simulink model "s0322"  (Simulink 7.0)
settings: Solver=ode3  SolverMode=SingleTasking  StartTime=0.0  StopTime=900  FixedStep=1  MaxStep=1  RelTol=1e-3  AbsTol=1e-6
values from neighbouring files (symbols this model uses):
  ITnnen = G.den{1}    [m0322.m]
  ITnzae = G.num{1}    [m0322.m]
  Kis = .5    (= 0.5)    [m0320.m]    (also in m0322.m = 0.6)
  nen = Gs.den{1}    [m0251.m]    (also in m0252.m; m0256.m; m0258.m; m0304.m = G.den{1})
  T1 = 3*T1    (= 0.3)    [m0203.m]    (also in m0204.m = 0.1; m0205.m = 0.1; m0207.m = 0.1; m0221d.m = 1/a0)
  Tt = .4    (= 0.4)    [m0108d.m]    (also in m0259.m = 1; m0314.m = 2.13; m0322.m = 0.8; m0326.m = 4)
  ydach = 1    [m0305.m]    (also in m0306.m; m0311.m; m0312b.m; m0313.m)
  zae = Gs.num{1}    [m0251.m]    (also in m0252.m; m0256.m; m0258.m; m0304.m = G.num{1})
settings Model: Creator=froriep  LastModifiedBy=froriep
settings DataIOCC: LimitDataPoints=off  SaveOutput=off  SaveTime=off
settings OptimizationCC: BooleanDataType=off  InlineInvariantSignals=on
settings DebuggingCC: SaveWithParameterizedLinksMsg=none  SignalResolutionControl=TryResolveAllWithWarning  SolverPrmCheckMsg=none  MultiTaskDSMMsg=warning  MultiTaskCondExecSysMsg=none  StrictBusMsg=None
settings HardwareCC: TargetUnknown=on
settings RTWCC: IncludeERTFirstTime=on
settings GRTTargetCC: TargetFcnLib=ansi_tfl_tmw.mat  ModelReferenceCompliant=off  MatFileLogging=off

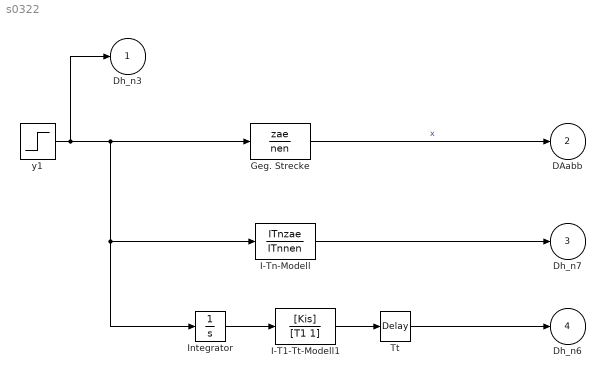
== system s0322 ==
  Geg. Strecke : TransferFcn  Numerator=zae  Denominator=nen
  I-T1-Tt-Modell1 : TransferFcn  Numerator=[Kis]  Denominator=[T1 1]
  I-Tn-Modell : TransferFcn  Numerator=ITnzae  Denominator=ITnnen
  Integrator : Integrator
  Tt : TransportDelay  DelayTime=Tt
  y1 : Step  Time=0  After=ydach  SampleTime=0
  Dh_n3 : Outport  OutDataType=sfix(16)  OutScaling=2^0
  DAabb : Outport  Port=2  OutDataType=sfix(16)  OutScaling=2^0
  Dh_n7 : Outport  Port=3  OutDataType=sfix(16)  OutScaling=2^0
  Dh_n6 : Outport  Port=4  OutDataType=sfix(16)  OutScaling=2^0
  wires:
  y1/1 -> Dh_n3/1, Geg. Strecke/1, I-Tn-Modell/1, Integrator/1
  Tt/1 -> Dh_n6/1
  I-Tn-Modell/1 -> Dh_n7/1
  Geg. Strecke/1 -> DAabb/1  "x"
  Integrator/1 -> I-T1-Tt-Modell1/1
  I-T1-Tt-Modell1/1 -> Tt/1
